simulink model "EPQ"  (R2018a)
settings: Solver=VariableStepAuto  StartTime=0.0  StopTime=10.0  RelTol=1e-3
libraries: aerolibutil x8, aerolibanim x2, simulink x2, vrlib x1, aerolibbdyn x1, aerolibatmos2 x1, sharedtransform x1, sharedutil x1
settings Model: Creator=rahul  LastModifiedBy=rahul

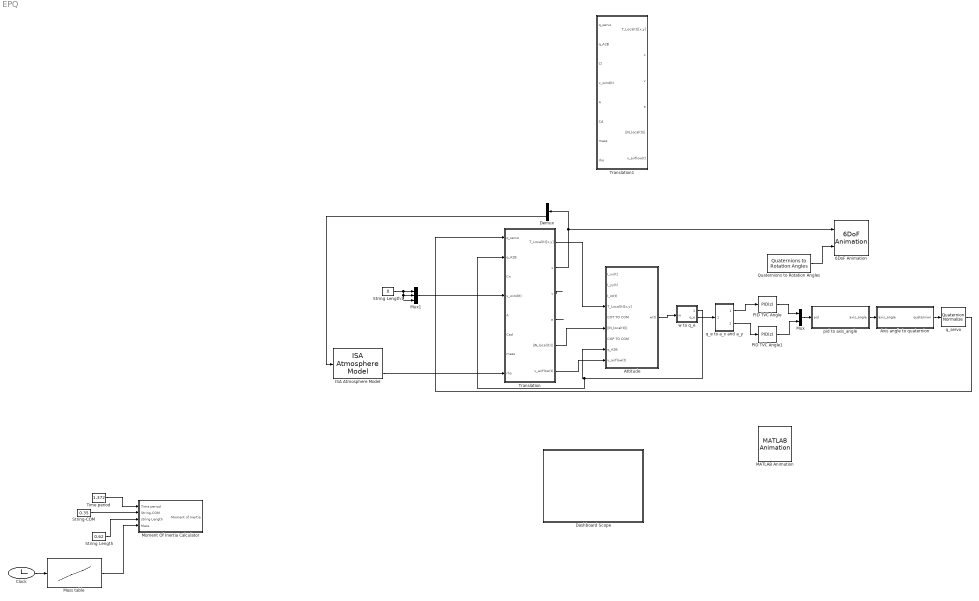
== system EPQ ==
  6DoF Animation : aerolibanim/6DoF Animation  u1=[0 4000 -2000 2000 -5000 -3000]  u2=0.1  u3=1.0  u4=[4000 0 -5000]  u5=Fly alongside  u6=[2000 500 -3150]  u7=10  u8=on
      settings: SourceProductName=Aerospace Blockset
  Attitude : Subsystem
  Axis angle to quaternion : MATLAB Function  TreatAsAtomicUnit=on
  Clock : Clock
  Dashboard Scope : Subsystem  DialogController=hmiCreateDDGDialog  IsWebBlock=on  mask(MWDashboardBlock){webBlockId=cd91c256-aca7-4cae-9769-d994bd04d296, webBlockType=sdiscope, ShowInitialText=on, HMISrcModelName=EPQ}
      mask prompts: webBlockId "WebBlock Id"; webBlockType "WebBlock Type"; HMISrcModelName "Source Model"
      mask help: SimulinkHMI:dialogs:HMIScopeDialogDesc
      mask Help: helpview([docroot '/mapfiles/simulink.map'], 'hmi_scope')
      mask Display:
      | if strcmp(get_param(bdroot(gcb),'BlockDiagramType'), 'library')
      |     image([(matlabroot) '/toolbox/simulink/hmi/icons/DashboardScope.png']);
      | end
  Demux : Demux  Outputs=3
  ISA Atmosphere Model : aerolibatmos2/ISA Atmosphere Model  custom=off  g=9.80665  gamma=1.4  R=287.0531  L=0.0065  h_trop=11000  h_strat=20000  rho0=1.225  P0=101325  T0=288.15  h0=0
      settings: SourceProductName=Aerospace Blockset
  MATLAB Animation : aerolibanim/MATLAB Animation  Tag=Matlab Animation 6 DOF  Vehicles=1  Geometries='astredwedge.mat'  BoundingBoxCoordinates=[-50,50,-50,50,-50,50]  CameraOffset=[-150,-50,0]  CameraViewAngle=3  SampleTime=0.2  FigurePosition=[393,293,295,206]
      settings: SourceProductName=Aerospace Blockset  SourceProductBaseCode=AE
  Mass table : Lookup  InputValues=[0,1]  Table=[0.975,.8]  LookUpMeth=Use Input Nearest  SaturateOnIntegerOverflow=on
  Moment Of Inertia Calculator : Subsystem
  Mux : Mux  Inputs=2
  Mux1 : Mux  Inputs=3
  PID TVC Angle : simulink/Continuous/PID Controller  Controller=PID  TimeDomain=Discrete-time  SampleTime=0.02  IntegratorMethod=Trapezoidal  FilterMethod=Trapezoidal  Form=Parallel  UseFilter=on  ControllerParametersSource=internal  P=0.0444910192906637  I=0.00251899563332339  D=0.170401833942346  N=91.5676010079333  InitialConditionSource=internal  InitialConditionForIntegrator=0  InitialConditionForFilter=0  ExternalReset=none  LimitOutput=on  UpperSaturationLimit=0.1745329252  LowerSaturationLimit=-0.1745329252  LinearizeAsGain=on  AntiWindupMode=none  Kb=1  TrackingMode=off  Kt=1  PParamMin=[]  PParamMax=[]  IParamMin=[]  IParamMax=[]  DParamMin=[]  DParamMax=[]  NParamMin=[]  NParamMax=[]  KbParamMin=[]  KbParamMax=[]  KtParamMin=[]  KtParamMax=[]  POutMin=[]  POutMax=[]  IOutMin=[]  IOutMax=[]  DOutMin=[]  DOutMax=[]  NOutMin=[]  NOutMax=[]  KbOutMin=[]  KbOutMax=[]  KtOutMin=[]  KtOutMax=[]  IntegratorOutMin=[]  IntegratorOutMax=[]  FilterOutMin=[]  FilterOutMax=[]  SumOutMin=[]  SumOutMax=[]  SumI1OutMin=[]  SumI1OutMax=[]  SumI2OutMin=[]  SumI2OutMax=[]  SumI3OutMin=[]  SumI3OutMax=[]  SumDOutMin=[]  SumDOutMax=[]  SaturationOutMin=[]  SaturationOutMax=[]  IntegratorContinuousStateAttributes=''  IntegratorStateMustResolveToSignalObject=off  IntegratorRTWStateStorageClass=Auto  FilterContinuousStateAttributes=''  FilterStateMustResolveToSignalObject=off  FilterRTWStateStorageClass=Auto  DifferentiatorICPrevScaledInput=0  DifferentiatorOutMin=[]  DifferentiatorOutMax=[]  FilterDiffOutCoefMin=[]  FilterDiffOutCoefMax=[]  SumDenOutMin=[]  SumDenOutMax=[]  SumNumOutMin=[]  SumNumOutMax=[]  ReciprocalOutMin=[]  ReciprocalOutMax=[]  DivideOutMin=[]  DivideOutMax=[]  TunerSelectOption=Transfer Function Based (PID Tuner App)
  PID TVC Angle1 : simulink/Continuous/PID Controller  Controller=PID  TimeDomain=Discrete-time  SampleTime=0.02  IntegratorMethod=Trapezoidal  FilterMethod=Trapezoidal  Form=Parallel  UseFilter=on  ControllerParametersSource=internal  P=0.0444910192906637  I=0.00251899563332339  D=0.170401833942346  N=91.5676010079333  InitialConditionSource=internal  InitialConditionForIntegrator=0  InitialConditionForFilter=0  ExternalReset=none  LimitOutput=on  UpperSaturationLimit=0.1745329252  LowerSaturationLimit=-0.1745329252  LinearizeAsGain=on  AntiWindupMode=none  Kb=1  TrackingMode=off  Kt=1  PParamMin=[]  PParamMax=[]  IParamMin=[]  IParamMax=[]  DParamMin=[]  DParamMax=[]  NParamMin=[]  NParamMax=[]  KbParamMin=[]  KbParamMax=[]  KtParamMin=[]  KtParamMax=[]  POutMin=[]  POutMax=[]  IOutMin=[]  IOutMax=[]  DOutMin=[]  DOutMax=[]  NOutMin=[]  NOutMax=[]  KbOutMin=[]  KbOutMax=[]  KtOutMin=[]  KtOutMax=[]  IntegratorOutMin=[]  IntegratorOutMax=[]  FilterOutMin=[]  FilterOutMax=[]  SumOutMin=[]  SumOutMax=[]  SumI1OutMin=[]  SumI1OutMax=[]  SumI2OutMin=[]  SumI2OutMax=[]  SumI3OutMin=[]  SumI3OutMax=[]  SumDOutMin=[]  SumDOutMax=[]  SaturationOutMin=[]  SaturationOutMax=[]  IntegratorContinuousStateAttributes=''  IntegratorStateMustResolveToSignalObject=off  IntegratorRTWStateStorageClass=Auto  FilterContinuousStateAttributes=''  FilterStateMustResolveToSignalObject=off  FilterRTWStateStorageClass=Auto  DifferentiatorICPrevScaledInput=0  DifferentiatorOutMin=[]  DifferentiatorOutMax=[]  FilterDiffOutCoefMin=[]  FilterDiffOutCoefMax=[]  SumDenOutMin=[]  SumDenOutMax=[]  SumNumOutMin=[]  SumNumOutMax=[]  ReciprocalOutMin=[]  ReciprocalOutMax=[]  DivideOutMin=[]  DivideOutMax=[]  TunerSelectOption=Transfer Function Based (PID Tuner App)
  Quaternions to Rotation Angles : sharedtransform/Quaternions to Rotation Angles  rotationOrder=ZYX  aMode=aMode
      settings: SourceProductBaseCode=AE
  String Length : Constant  Value=0.62
  String Length1 : Constant  Value=0
  String-COM : Constant  Value=0.35
  Time period : Constant  Value=1.372
  Translation : Subsystem
  Translation1 : Subsystem
  pid to axis_angle : MATLAB Function  TreatAsAtomicUnit=on
  q_e to a_x and a_y : Subsystem
  q_servo : sharedutil/Quaternion Normalize  aMode=aMode
      settings: SourceProductName=Aerospace Blockset  SourceProductBaseCode=AE
  w to q_e : Subsystem
  wires:
  String Length/1 -> Moment Of Inertia Calculator/3(string Length)
  Mass table/1 -> Moment Of Inertia Calculator/4(Mass)
  Time period/1 -> Moment Of Inertia Calculator/1(Time period)
  Clock/1 -> Mass table/1
  String-COM/1 -> Moment Of Inertia Calculator/2(String-COM)
  Translation/5(||N_local(t)||) -> Attitude/6(||N_local(t)||)
  Translation/6(v_airflow(t)) -> Attitude/9(v_airflow(t))
  Translation/1(T_Local(t)[x,y]) -> Attitude/4(T_Local(t)[x,y])
  Translation/2(x) -> 6DoF Animation/1, Demux/1
  Translation/3(v) -> ?
  Translation/4(a) -> ?
  Quaternions to Rotation Angles/1 -> 6DoF Animation/2
  Axis angle to quaternion/1(quaternion) -> q_servo/1
  pid to axis_angle/1(axis_angle) -> Axis angle to quaternion/1(axis_angle)
  PID TVC Angle/1 -> Mux/1
  PID TVC Angle1/1 -> Mux/2
  Attitude/1(w(t)) -> w to q_e/1(w)
  w to q_e/2(q_e) -> q_e to a_x and a_y/1(q_e)
  q_e to a_x and a_y/1(a_x) -> PID TVC Angle/1
  q_e to a_x and a_y/2(a_y) -> PID TVC Angle1/1
  Mux/1 -> pid to axis_angle/1(pid)
  q_servo/1 -> Translation/1(q_servo)
  w to q_e/1(q_A2B) -> Translation/2(q_A2B), Attitude/8(q_A2B)
  ISA Atmosphere Model/4 -> Translation/8(rho)
  Demux/3 -> ISA Atmosphere Model/1
  Mux1/1 -> Translation/4(v_wind(t))
  String Length1/1 -> Mux1/1, Mux1/2, Mux1/3

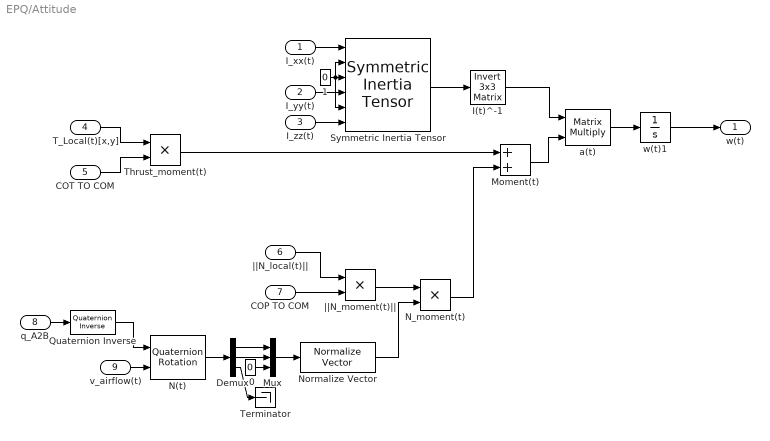
== system EPQ/Attitude ==
  I_xx(t) : Inport
  I_yy(t) : Inport  Port=2
  I_zz(t) : Inport  Port=3
  T_Local(t)[x,y] : Inport  Port=4
  COT TO COM : Inport  Port=5
  ||N_local(t)|| : Inport  Port=6
  COP TO COM : Inport  Port=7
  q_A2B : Inport  Port=8
  v_airflow(t) : Inport  Port=9
  0 : Constant  Value=0
  1 : Constant  Value=0
  Demux : Demux  Outputs=3
  I(t)^-1 : aerolibutil/Invert  3x3 Matrix
  Moment(t) : Sum
  Mux : Mux  Inputs=3
  N(t) : aerolibutil/Quaternion Rotation
  N_moment(t) : Product
  Normalize Vector : vrlib/Utilities/Normalize Vector  maxzero=0
      settings: SourceProductName=Simulink 3D Animation  SourceProductBaseCode=VR
  Quaternion Inverse : aerolibutil/Quaternion Inverse
      settings: SourceProductName=Aerospace Blockset
  Symmetric Inertia Tensor : aerolibbdyn/Symmetric Inertia Tensor
      settings: SourceProductName=Aerospace Blockset  SourceProductBaseCode=AE
  Terminator : Terminator
  Thrust_moment(t) : Product
  a(t) : Product  Multiplication=Matrix(*)
  w(t)1 : Integrator
  ||N_moment(t)|| : Product
  w(t) : Outport
  wires:
  Thrust_moment(t)/1 -> Moment(t)/1
  I_yy(t)/1 -> Symmetric Inertia Tensor/4
  COT TO COM/1 -> Thrust_moment(t)/2
  I_xx(t)/1 -> Symmetric Inertia Tensor/1
  Demux/2 -> Mux/2
  T_Local(t)[x,y]/1 -> Thrust_moment(t)/1
  I(t)^-1/1 -> a(t)/1
  COP TO COM/1 -> ||N_moment(t)||/2
  v_airflow(t)/1 -> N(t)/2
  Demux/1 -> Mux/1
  N(t)/1 -> Demux/1
  I_zz(t)/1 -> Symmetric Inertia Tensor/6
  w(t)1/1 -> w(t)/1
  0/1 -> Mux/3
  Mux/1 -> Normalize Vector/1
  N_moment(t)/1 -> Moment(t)/2
  ||N_moment(t)||/1 -> N_moment(t)/1
  a(t)/1 -> w(t)1/1
  q_A2B/1 -> Quaternion Inverse/1
  Moment(t)/1 -> a(t)/2
  Symmetric Inertia Tensor/1 -> I(t)^-1/1
  Normalize Vector/1 -> N_moment(t)/2
  ||N_local(t)||/1 -> ||N_moment(t)||/1
  1/1 -> Symmetric Inertia Tensor/2, Symmetric Inertia Tensor/3, Symmetric Inertia Tensor/5
  Quaternion Inverse/1 -> N(t)/1
  Demux/3 -> Terminator/1

== system EPQ/Dashboard Scope ==

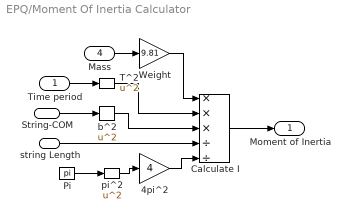
== system EPQ/Moment Of Inertia Calculator ==
  Time period : Inport
  String-COM : Inport  Port=2
  string Length : Inport  Port=3
  Mass : Inport  Port=4
  4pi^2 : Gain  Gain=4
  Calculate I : Product  Inputs=***//
  Pi : Constant  Value=pi
  T^2 : Math  Operator=square  SaturateOnIntegerOverflow=on
  Weight : Gain  Gain=9.81
  b^2 : Math  Operator=square  SaturateOnIntegerOverflow=on
  pi^2 : Math  Operator=square  SaturateOnIntegerOverflow=on
  Moment of Inertia : Outport
  wires:
  Time period/1 -> T^2/1
  Calculate I/1 -> Moment of Inertia/1
  string Length/1 -> Calculate I/4
  Mass/1 -> Weight/1
  Weight/1 -> Calculate I/1
  pi^2/1 -> 4pi^2/1
  b^2/1 -> Calculate I/3
  T^2/1 -> Calculate I/2
  String-COM/1 -> b^2/1
  Pi/1 -> pi^2/1
  4pi^2/1 -> Calculate I/5

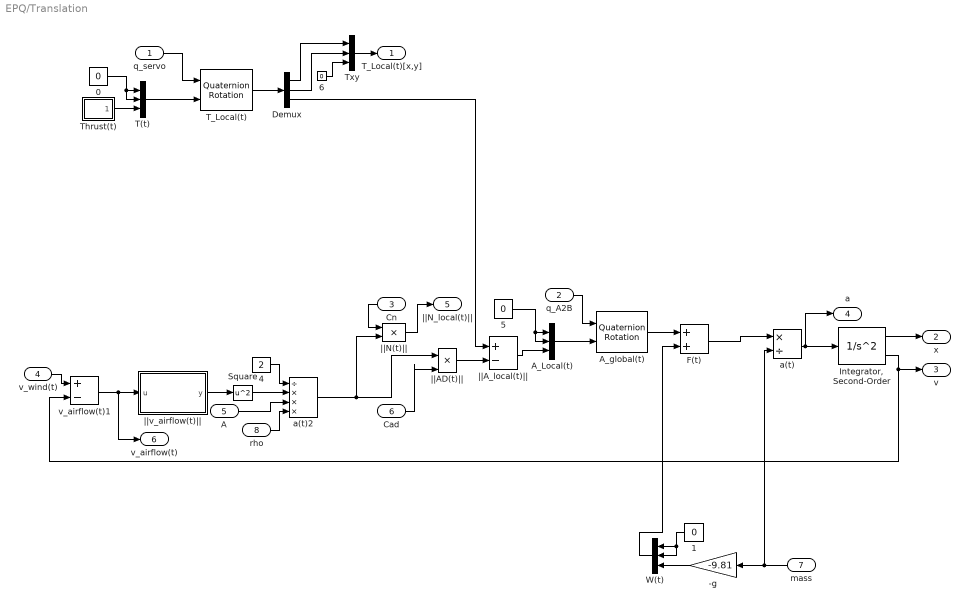
== system EPQ/Translation ==
  q_servo : Inport
  q_A2B : Inport  Port=2
  Cn : Inport  Port=3
  v_wind(t) : Inport  Port=4
  A : Inport  Port=5
  Cad : Inport  Port=6
  mass : Inport  Port=7
  rho : Inport  Port=8
  -g : Gain  Gain=-9.81
  {0..1,5..6} (4 alike) : Constant  Value=0
  4 : Constant  Value=2
  A_Local(t) : Mux  Inputs=3
  A_global(t) : aerolibutil/Quaternion Rotation
  Demux : Demux  Outputs=3
  F(t) : Sum
  "Integrator, Second-Order" : SecondOrderIntegrator  LimitX=on  LowerLimitX=0
  Square : Math  Operator=square  SaturateOnIntegerOverflow=on
  T(t) : Mux  Inputs=3
  T_Local(t) : aerolibutil/Quaternion Rotation
  Thrust(t) : Subsystem
  Txy : Mux  Inputs=3
  W(t) : Mux  Inputs=3
  a(t) : Product  Inputs=*/
  a(t)2 : Product  Inputs=/***
  v_airflow(t)1 : Sum  Inputs=+-
  ||AD(t)|| : Product  Inputs=**
  ||A_local(t)|| : Sum  Inputs=+-
  ||N(t)|| : Product  Inputs=**
  ||v_airflow(t)|| : MATLAB Function  TreatAsAtomicUnit=on
  T_Local(t)[x,y] : Outport
  x : Outport  Port=2
  v : Outport  Port=3
  a : Outport  Port=4
  ||N_local(t)|| : Outport  Port=5
  v_airflow(t) : Outport  Port=6
  wires:
  "Integrator, Second-Order"/1 -> x/1
  v_airflow(t)1/1 -> ||v_airflow(t)||/1(u), v_airflow(t)/1
  T_Local(t)/1 -> Demux/1
  A_Local(t)/1 -> A_global(t)/2
  Square/1 -> a(t)2/2
  a(t)/1 -> a/1, "Integrator, Second-Order"/1
  q_servo/1 -> T_Local(t)/1
  A_global(t)/1 -> F(t)/1
  F(t)/1 -> a(t)/1
  -g/1 -> W(t)/3
  A/1 -> a(t)2/3
  v_wind(t)/1 -> v_airflow(t)1/1
  "Integrator, Second-Order"/2 -> v/1, v_airflow(t)1/2
  1/1 -> W(t)/1, W(t)/2
  a(t)2/1 -> ||AD(t)||/1, ||N(t)||/2
  W(t)/1 -> F(t)/2
  ||A_local(t)||/1 -> A_Local(t)/3
  ||v_airflow(t)||/1(y) -> Square/1
  T(t)/1 -> T_Local(t)/2
  4/1 -> a(t)2/1
  Txy/1 -> T_Local(t)[x,y]/1
  Demux/1 -> Txy/1
  5/1 -> A_Local(t)/2, A_Local(t)/1
  Thrust(t)/1(Thrust) -> T(t)/3
  Demux/2 -> Txy/2
  q_A2B/1 -> A_global(t)/1
  0/1 -> T(t)/2, T(t)/1
  mass/1 -> a(t)/2, -g/1
  Demux/3 -> ||A_local(t)||/1
  6/1 -> Txy/3
  Cn/1 -> ||N(t)||/1
  ||N(t)||/1 -> ||N_local(t)||/1
  Cad/1 -> ||AD(t)||/2
  rho/1 -> a(t)2/4
  ||AD(t)||/1 -> ||A_local(t)||/2

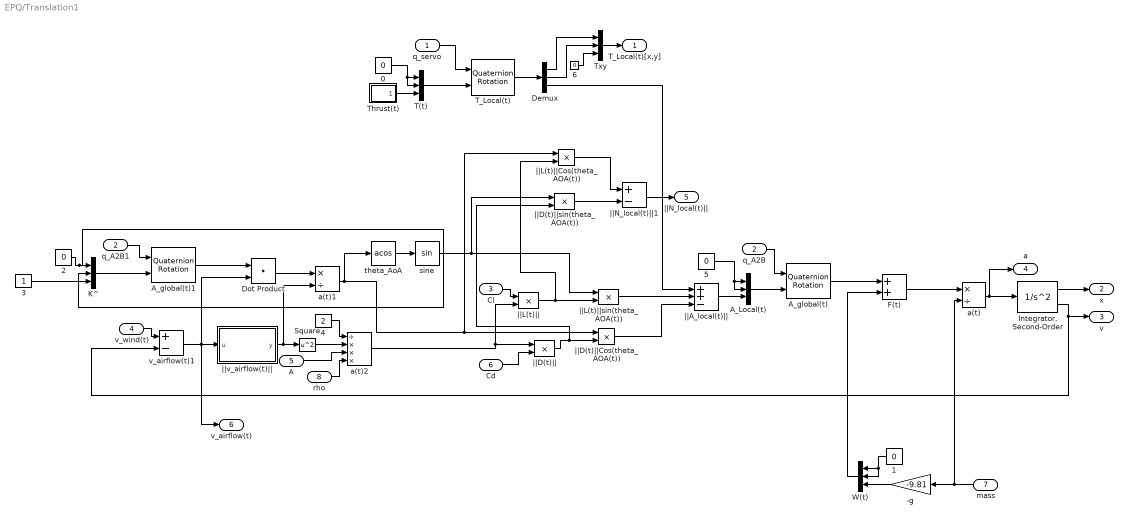
== system EPQ/Translation1 ==
  q_servo : Inport
  q_A2B : Inport  Port=2
  Cl : Inport  Port=3
  v_wind(t) : Inport  Port=4
  A : Inport  Port=5
  Cd : Inport  Port=6
  mass : Inport  Port=7
  rho : Inport  Port=8
  -g : Gain  Gain=-9.81
  {0..2,5..6} (5 alike) : Constant  Value=0
  3 : Constant
  4 : Constant  Value=2
  A_Local(t) : Mux  Inputs=3
  A_global(t) : aerolibutil/Quaternion Rotation
  A_global(t)1 : aerolibutil/Quaternion Rotation
  Demux : Demux  Outputs=3
  Dot Product : DotProduct  InputSameDT=on  OutDataTypeStr=Inherit: Inherit via internal rule
  F(t) : Sum
  "Integrator, Second-Order" : SecondOrderIntegrator  LimitX=on  LowerLimitX=0
  K^ : Mux  Inputs=3
  Square : Math  Operator=square  SaturateOnIntegerOverflow=on
  T(t) : Mux  Inputs=3
  T_Local(t) : aerolibutil/Quaternion Rotation
  Thrust(t) : Subsystem
  Txy : Mux  Inputs=3
  W(t) : Mux  Inputs=3
  a(t) : Product  Inputs=*/
  a(t)1 : Product  Inputs=*/
  a(t)2 : Product  Inputs=/***
  q_A2B1 : InportShadow  Port=2
  sine : Trigonometry
  theta_AoA : Trigonometry  Operator=acos
  v_airflow(t)1 : Sum  Inputs=+-
  ||A_local(t)|| : Sum  Inputs=++-
  ||D(t)|| : Product  Inputs=**
  ||D(t)||Cos(theta_AOA(t)) : Product  Inputs=**
  ||D(t)||sin(theta_AOA(t)) : Product  Inputs=**
  ||L(t)|| : Product  Inputs=**
  ||L(t)||Cos(theta_AOA(t)) : Product  Inputs=**
  ||L(t)||sin(theta_AOA(t)) : Product  Inputs=**
  ||N_local(t)||1 : Sum  Inputs=+-
  ||v_airflow(t)|| : MATLAB Function  TreatAsAtomicUnit=on
  T_Local(t)[x,y] : Outport
  x : Outport  Port=2
  v : Outport  Port=3
  a : Outport  Port=4
  ||N_local(t)|| : Outport  Port=5
  v_airflow(t) : Outport  Port=6
  wires:
  "Integrator, Second-Order"/1 -> x/1
  v_airflow(t)1/1 -> Dot Product/2, ||v_airflow(t)||/1(u), v_airflow(t)/1
  T_Local(t)/1 -> Demux/1
  3/1 -> K^/3
  A_Local(t)/1 -> A_global(t)/2
  K^/1 -> A_global(t)1/2
  Square/1 -> a(t)2/2
  a(t)/1 -> a/1, "Integrator, Second-Order"/1
  q_servo/1 -> T_Local(t)/1
  A_global(t)/1 -> F(t)/1
  F(t)/1 -> a(t)/1
  -g/1 -> W(t)/3
  theta_AoA/1 -> sine/1
  A/1 -> a(t)2/3
  a(t)1/1 -> ||L(t)||Cos(theta_AOA(t))/1, ||D(t)||Cos(theta_AOA(t))/1, theta_AoA/1
  v_wind(t)/1 -> v_airflow(t)1/1
  "Integrator, Second-Order"/2 -> v/1, v_airflow(t)1/2
  Dot Product/1 -> a(t)1/1
  2/1 -> K^/2, K^/1
  1/1 -> W(t)/1, W(t)/2
  a(t)2/1 -> ||L(t)||/2, ||D(t)||/1
  W(t)/1 -> F(t)/2
  ||A_local(t)||/1 -> A_Local(t)/3
  ||v_airflow(t)||/1(y) -> a(t)1/2, Square/1
  T(t)/1 -> T_Local(t)/2
  4/1 -> a(t)2/1
  Txy/1 -> T_Local(t)[x,y]/1
  Demux/1 -> Txy/1
  5/1 -> A_Local(t)/2, A_Local(t)/1
  A_global(t)1/1 -> Dot Product/1
  Thrust(t)/1(Thrust) -> T(t)/3
  Demux/2 -> Txy/2
  q_A2B/1 -> A_global(t)/1
  0/1 -> T(t)/2, T(t)/1
  mass/1 -> a(t)/2, -g/1
  Demux/3 -> ||A_local(t)||/1
  q_A2B1/1 -> A_global(t)1/1
  6/1 -> Txy/3
  Cl/1 -> ||L(t)||/1
  ||L(t)||sin(theta_AOA(t))/1 -> ||A_local(t)||/2
  ||L(t)||/1 -> ||L(t)||Cos(theta_AOA(t))/2, ||L(t)||sin(theta_AOA(t))/2
  sine/1 -> ||D(t)||sin(theta_AOA(t))/1, ||L(t)||sin(theta_AOA(t))/1
  Cd/1 -> ||D(t)||/2
  ||D(t)||/1 -> ||D(t)||sin(theta_AOA(t))/2, ||D(t)||Cos(theta_AOA(t))/2
  ||D(t)||Cos(theta_AOA(t))/1 -> ||A_local(t)||/3
  ||L(t)||Cos(theta_AOA(t))/1 -> ||N_local(t)||1/1
  ||D(t)||sin(theta_AOA(t))/1 -> ||N_local(t)||1/2
  ||N_local(t)||1/1 -> ||N_local(t)||/1
  rho/1 -> a(t)2/4

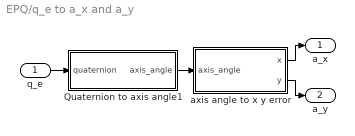
== system EPQ/q_e to a_x and a_y ==
  q_e : Inport
  Quaternion to axis angle1 : MATLAB Function  TreatAsAtomicUnit=on
  axis angle to x y error : MATLAB Function  TreatAsAtomicUnit=on
  a_x : Outport
  a_y : Outport  Port=2
  wires:
  Quaternion to axis angle1/1(axis_angle) -> axis angle to x y error/1(axis_angle)
  axis angle to x y error/1(x) -> a_x/1
  axis angle to x y error/2(y) -> a_y/1
  q_e/1 -> Quaternion to axis angle1/1(quaternion)

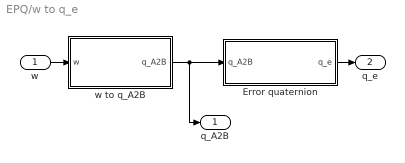
== system EPQ/w to q_e ==
  w : Inport
  Error quaternion : MATLAB Function  TreatAsAtomicUnit=on
  w to q_A2B : MATLAB Function  TreatAsAtomicUnit=on
  q_A2B : Outport
  q_e : Outport  Port=2
  wires:
  w/1 -> w to q_A2B/1(w)
  w to q_A2B/1(q_A2B) -> q_A2B/1, Error quaternion/1(q_A2B)
  Error quaternion/1(q_e) -> q_e/1

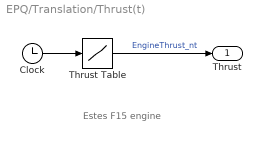
== system EPQ/Translation/Thrust(t) ==
  note: Estes F15 engine
  Clock : Clock
  Thrust Table : Lookup  InputValues=|  Table=[0,12.5,25,16.5,15.25,15,14.5,14.5,14.25,14,13,13,0]  LookUpMeth=Interpolation-Use End Values  SaturateOnIntegerOverflow=on
      | [0,
      | 0.25,
      | 0.5,
      | 0.75,
      | 1,
      | 1.25,
      | 1.5,
      | 2,
      | 2.25,
      | 2.5,
      | 3,
      | 3.25,
      | 3.5]
  Thrust : Outport
  wires:
  Clock/1 -> Thrust Table/1
  Thrust Table/1 -> Thrust/1  "EngineThrust_nt"

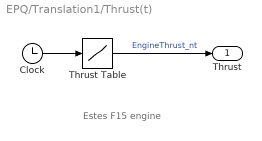
== system EPQ/Translation1/Thrust(t) ==
  note: Estes F15 engine
  Clock : Clock
  Thrust Table : Lookup  InputValues=|  Table=[0,12.5,25,16.5,15.25,15,14.5,14.5,14.25,14,13,13,0]  LookUpMeth=Interpolation-Use End Values  SaturateOnIntegerOverflow=on
      | [0,
      | 0.25,
      | 0.5,
      | 0.75,
      | 1,
      | 1.25,
      | 1.5,
      | 2,
      | 2.25,
      | 2.5,
      | 3,
      | 3.25,
      | 3.5]
  Thrust : Outport
  wires:
  Clock/1 -> Thrust Table/1
  Thrust Table/1 -> Thrust/1  "EngineThrust_nt"

== matlab function EPQ/w to q_e/Error quaternion ==
  data: q_A2B input; q_e output
function q_e = fcn(q_A2B)

if abs(q_A2B(1)) ~= 1
    theta = acos(q_A2B(1));
    x = atan(tan(theta) * q_A2B(4)/sin(theta));
    roll = [cos(x), 0, 0,sin(x)];
    q_e = quatmultiply(quatinv(q_A2B), roll);
    t = acos(q_e(1));
    if t < 0
        q_e(1) = cos(pi - t);
    end
    %if t < -pi/2
        %error(1) = cos(t + pi); %if more than -180 degree rotation add 360 degrees to angle, only pi as q0 is divided by 2
    %elseif t > pi/2
        %error(1) = cos(t - pi); %if more than 180 degree rotation subtract 360 degrees to angle, only pi as q0 is divided by 2
    %end
else
    q_e = [1, 0, 0, 0];
end

== matlab function EPQ/Translation/||v_airflow(t)|| ==
  data: u input; y output
function y = VectorNorm(u)

y = norm(u);

== matlab function EPQ/w to q_e/w to q_A2B ==
  data: w input; q_A2B output
function q_A2B = fcn(w)
persistent q_A2B_prev

if isempty(q_A2B_prev)
    q_A2B_prev = [1 0 0 0];
end

W = [0 w];
q_A2Bdot = quatmultiply(dt/2 * W, q_A2B_prev);
q_A2B = quatnormalize(q_A2B_prev + q_A2Bdot);
q_A2B_prev = q_A2B;

== matlab function EPQ/Axis angle to quaternion ==
  data: axis_angle input; quaternion output
function quaternion = fcn(axis_angle)

angle = axis_angle(1)/2;
sine = sin(angle);
quaternion = [cos(angle); sine * axis_angle(2); sine * axis_angle(3); sine * axis_angle(4)];

== matlab function EPQ/q_e to a_x and a_y/Quaternion to axis angle1 ==
  settings: updateMethod=DISCRETE
  data: quaternion input; axis_angle output
function axis_angle = fcn(quaternion)

persistent previous_axis_vector;

if abs(quaternion(1)) == 1
    angle = 0; %if 0 degree rotation dont divide by 0 http://www.euclideanspace.com/maths/geometry/rotations/conversions/quaternionToAngle/ 
else
    s = (1-quaternion(1)^2)^0.5;
    previous_axis_vector = [quaternion(2) quaternion(3) quaternion(4)] / s;
    angle = 2 * acos(quaternion(1));
end

if isempty(previous_axis_vector)
    previous_axis_vector = [1 0 0];
end

axis_angle = [angle previous_axis_vector];

== matlab function EPQ/q_e to a_x and a_y/axis angle to x y error ==
  settings: updateMethod=DISCRETE
  data: axis_angle input; x output; y output
function [x,y] = fcn(axis_angle)

y= axis_angle(1) * axis_angle(2);
x= axis_angle(1) * axis_angle(3);

== matlab function EPQ/pid to axis_angle ==
  settings: updateMethod=DISCRETE
  data: pid input; axis_angle output
function axis_angle = fcn(pid)

angle = norm(pid);
if angle == 0
    v = [1 0];
else
    v = [pid(1)/angle pid(2)/angle];
end
axis_angle = [angle v 0];

== matlab function EPQ/Translation1/||v_airflow(t)|| ==
  data: u input; y output
function y = VectorNorm(u)

y = norm(u);
